simulink model "stateFeedbackIntegralControl"  (R2024b)
settings: Solver=VariableStepAuto  StartTime=0.0  StopTime=10.0  RelTol=1e-3
values from neighbouring files (symbols this model uses):
  A = zeros(4)    [me_577_final_project_main.m]
  B = zeros(4,1)    [me_577_final_project_main.m]
  C = eye(4)    [me_577_final_project_main.m]
  cartPosition = 5    [me_577_final_project_main.m]
  D = zeros(4, 1)    [me_577_final_project_main.m]
  impulseAmp = 0    [me_577_final_project_main.m]
  K = gainMatrix(1:4)    [me_577_final_project_main.m]
  KI = -gainMatrix(5)    [me_577_final_project_main.m]
  periodicDisturbanceAmp = 100    [me_577_final_project_main.m]
  periodicDisturbanceFreq = 10    [me_577_final_project_main.m]
settings Model: Creator=cory  LastModifiedBy=cgobl

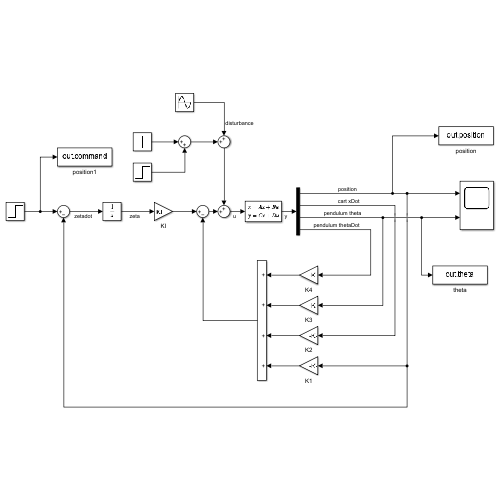
[thumbnail: Simulink's stored preview of the top-level diagram]
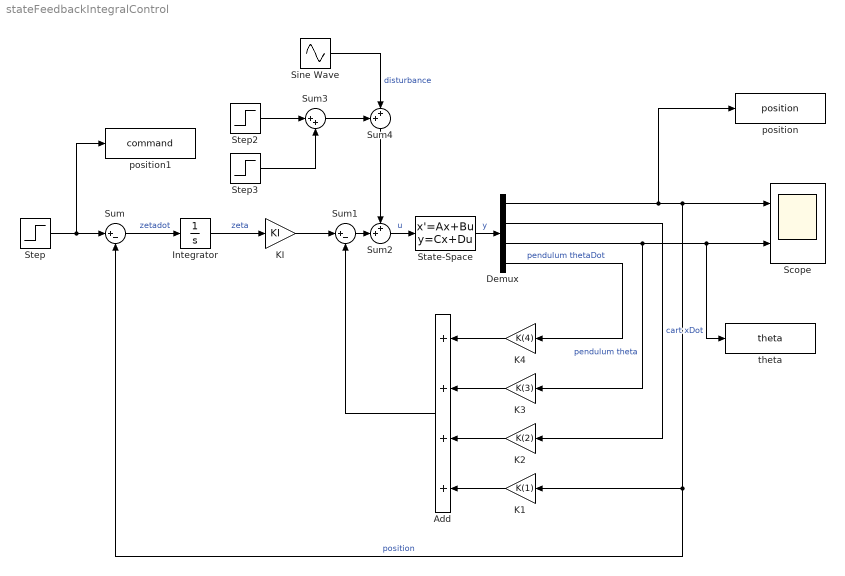
== system stateFeedbackIntegralControl ==
  Add : Sum  Inputs=++++
  Demux : Demux
  Integrator : Integrator
  K1 : Gain  Gain=K(1)
  K2 : Gain  Gain=K(2)
  K3 : Gain  Gain=K(3)
  K4 : Gain  Gain=K(4)
  KI : Gain  Gain=KI
  Scope : Scope  NumInputPorts=2
  Sine Wave : Sin  Amplitude=periodicDisturbanceAmp  Frequency=periodicDisturbanceFreq  SampleTime=0
  State-Space : StateSpace  A=A  B=B  C=C  D=D  InitialCondition=0  ContinuousStateAttributes=['position','velocity','angle','omega']
  Step : Step  After=cartPosition  SampleTime=0
  Step2 : Step  Time=2  After=impulseAmp  SampleTime=0
  Step3 : Step  Time=2.5  After=-impulseAmp  SampleTime=0
  Sum : Sum  Inputs=|+-
  Sum1 : Sum  Inputs=|+-
  Sum2 : Sum  Inputs=++|
  Sum3 : Sum  Inputs=|++
  Sum4 : Sum  Inputs=++|
  position : ToWorkspace  VariableName=position  SampleTime=-1
      settings: Save2DSignal=2-D array (concatenate along first dimension)
  position1 : ToWorkspace  VariableName=command  SampleTime=-1
      settings: Save2DSignal=2-D array (concatenate along first dimension)
  theta : ToWorkspace  VariableName=theta  SampleTime=-1
      settings: Save2DSignal=2-D array (concatenate along first dimension)
  wires:
  Step/1 -> position1/1, Sum/1
  Sum/1 -> Integrator/1  "zetadot"
  Integrator/1 -> KI/1  "zeta"
  KI/1 -> Sum1/1
  Sum1/1 -> Sum2/2
  State-Space/1 -> Demux/1  "y"
  Demux/4 -> K4/1  "pendulum thetaDot"
  Demux/3 -> theta/1, Scope/2, K3/1  "pendulum theta"
  Demux/2 -> K2/1  "cart xDot"
  Demux/1 -> position/1, K1/1, Sum/2, Scope/1  "position"
  K4/1 -> Add/1
  K3/1 -> Add/2
  K2/1 -> Add/3
  K1/1 -> Add/4
  Add/1 -> Sum1/2
  Sum2/1 -> State-Space/1  "u"
  Step2/1 -> Sum3/1
  Step3/1 -> Sum3/2
  Sine Wave/1 -> Sum4/2  "disturbance"
  Sum4/1 -> Sum2/1
  Sum3/1 -> Sum4/1
